simulink model "lunarMissionModel"  (R2022b)
settings: Solver=ode45  StartTime=0.0  StopTime=tf  RelTol=1e-12  AbsTol=1e-12
undefined symbols (not defined in the file): burnDuration, deltaVDRODeparture, deltaVDROInsertion, deltaVOPF, deltaVRPF, DRODepartureDirection, DROInsertionDirection, km, OPFDirection, RPFDirection, s, tDRODeparture, tDROInsertion, tOPF, tRPF
libraries: aerolibcelestial x1, aerolibconvert2 x1
settings Model: Creator=hsaranat  LastModifiedBy=hsaranat
settings SolverCC: AutoScaleAbsTol=off

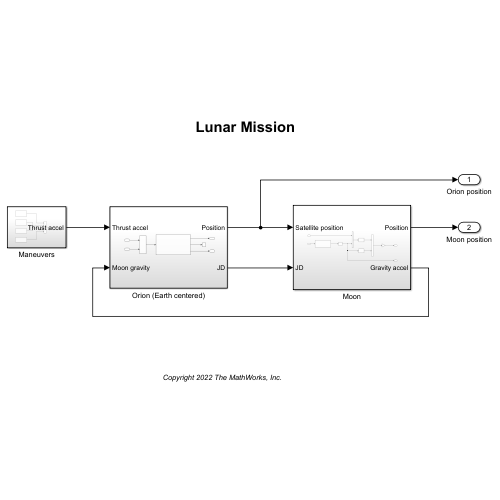
[thumbnail: Simulink's stored preview of the top-level diagram]
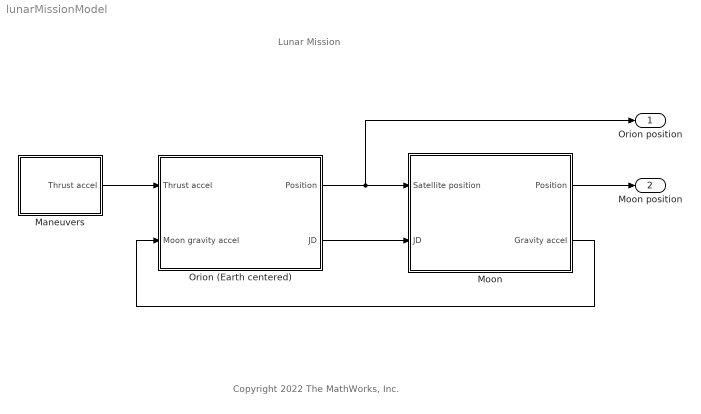
== system lunarMissionModel ==
  note: Lunar Mission
  note: Copyright 2022 The MathWorks, Inc.
  Maneuvers : Subsystem
  Moon : Subsystem
  Orion (Earth centered) : Subsystem
  Orion position : Outport
  Moon position : Outport  Port=2
  wires:
  Moon/1(Position) -> Moon position/1
  Orion (Earth centered)/2(JD) -> Moon/2(JD)
  Orion (Earth centered)/1(Position) -> Moon/1(Satellite position), Orion position/1
  Moon/2(Gravity accel) -> Orion (Earth centered)/2(Moon gravity accel)
  Maneuvers/1(Thrust accel) -> Orion (Earth centered)/1(Thrust accel)

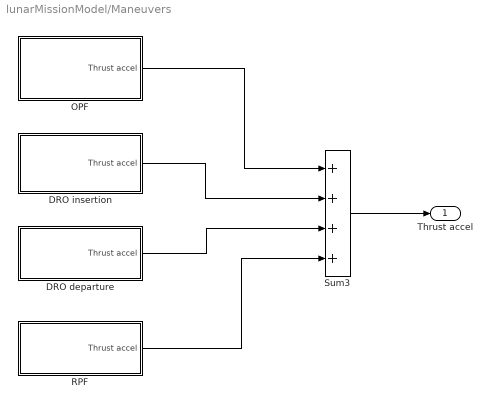
== system lunarMissionModel/Maneuvers ==
  DRO departure : Subsystem
  DRO insertion : Subsystem
  OPF : Subsystem
  RPF : Subsystem
  Sum3 : Sum  Inputs=++++
  Thrust accel : Outport
  wires:
  Sum3/1 -> Thrust accel/1
  OPF/1(Thrust accel) -> Sum3/1
  DRO insertion/1(Thrust accel) -> Sum3/2
  DRO departure/1(Thrust accel) -> Sum3/3
  RPF/1(Thrust accel) -> Sum3/4

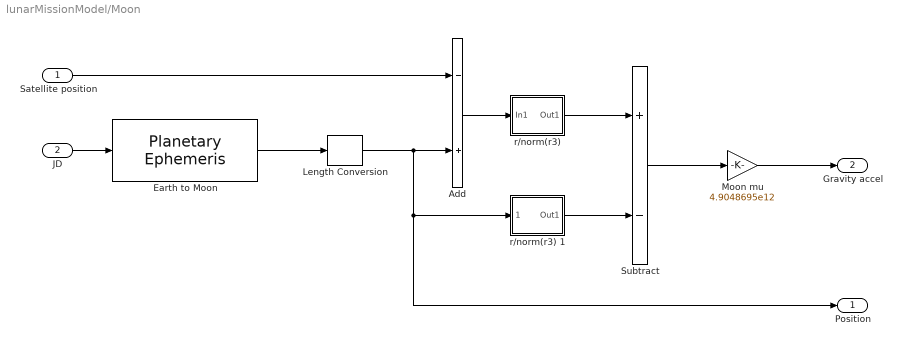
== system lunarMissionModel/Moon ==
  Satellite position : Inport
  JD : Inport  Port=2
  Add : Sum  Inputs=-+
  Earth to Moon : aerolibcelestial/Planetary Ephemeris  kmflag=km,km/s  epochflag=Julian date  de=DE405  nCenter=Earth  nTarget=Moon  errorflag=Error  velflag=off
  Length Conversion : aerolibconvert2/Length Conversion  IU=km  OU=m
  Moon mu : Gain  Gain=4.9048695e12
  Subtract : Sum  Inputs=+-
  r/norm(r3) : Subsystem
  r/norm(r3) 1 : Subsystem
  Position : Outport
  Gravity accel : Outport  Port=2
  wires:
  Earth to Moon/1 -> Length Conversion/1
  JD/1 -> Earth to Moon/1
  Length Conversion/1 -> Position/1, r/norm(r3) 1/1(1), Add/2
  r/norm(r3)/1(Out1) -> Subtract/1
  Moon mu/1 -> Gravity accel/1
  Satellite position/1 -> Add/1
  Add/1 -> r/norm(r3)/1(In1)
  r/norm(r3) 1/1(Out1) -> Subtract/2
  Subtract/1 -> Moon mu/1

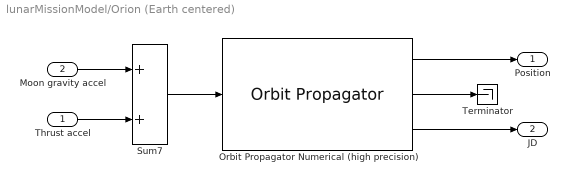
== system lunarMissionModel/Orion (Earth centered) ==
  Thrust accel : Inport
  Moon gravity accel : Inport  Port=2
  Orbit Propagator Numerical (high precision) : OrbitPropagator  propagator=Numerical (high precision)  accelIn=on  startDate=jd  action=None  stateFormatNum=ICRF state vector  eccentricity=0  inclination=30  raan=0  argPeriapsis=0  trueAnomaly=0  inertialPosition=initialPosition  inertialVelocity=initialVelocity  fixedPosition=[-4142689.0 -2676864.7 -4669861.6]  fixedVelocity=[1452.7 -6720.7 2568.1]  gravityModel=Point-mass  customR=3396200  customMu=4.305e13  customJ2=1.0826269e-03  customOmega=4.06125949e-3  useEOPs=off
  Sum7 : Sum
  Terminator : Terminator
  Position : Outport
  JD : Outport  Port=2
  wires:
  Orbit Propagator Numerical (high precision)/1 -> Position/1
  Orbit Propagator Numerical (high precision)/2 -> Terminator/1
  Sum7/1 -> Orbit Propagator Numerical (high precision)/1
  Orbit Propagator Numerical (high precision)/3 -> JD/1
  Thrust accel/1 -> Sum7/2
  Moon gravity accel/1 -> Sum7/1

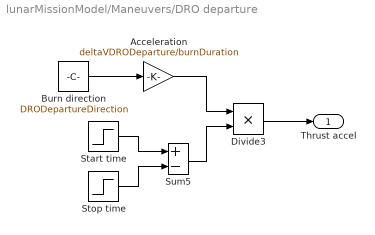
== system lunarMissionModel/Maneuvers/DRO departure ==
  Acceleration : Gain  Gain=deltaVDRODeparture/burnDuration
  Burn direction : Constant  Value=DRODepartureDirection
  Divide3 : Product  Inputs=**
  Start time : Step  Time=tDRODeparture  SampleTime=0
  Stop time : Step  Time=tDRODeparture+burnDuration  SampleTime=0
  Sum5 : Sum  Inputs=+-
  Thrust accel : Outport
  wires:
  Stop time/1 -> Sum5/2
  Burn direction/1 -> Acceleration/1
  Acceleration/1 -> Divide3/1
  Sum5/1 -> Divide3/2
  Start time/1 -> Sum5/1
  Divide3/1 -> Thrust accel/1

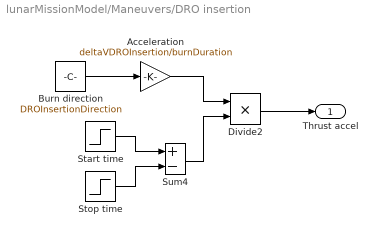
== system lunarMissionModel/Maneuvers/DRO insertion ==
  Acceleration : Gain  Gain=deltaVDROInsertion/burnDuration
  Burn direction : Constant  Value=DROInsertionDirection
  Divide2 : Product  Inputs=**
  Start time : Step  Time=tDROInsertion  SampleTime=0
  Stop time : Step  Time=tDROInsertion+burnDuration  SampleTime=0
  Sum4 : Sum  Inputs=+-
  Thrust accel : Outport
  wires:
  Acceleration/1 -> Divide2/1
  Start time/1 -> Sum4/1
  Divide2/1 -> Thrust accel/1
  Stop time/1 -> Sum4/2
  Sum4/1 -> Divide2/2
  Burn direction/1 -> Acceleration/1

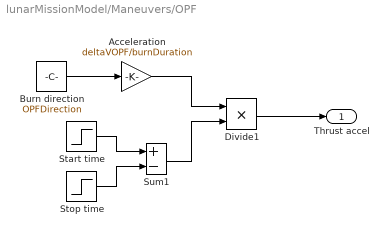
== system lunarMissionModel/Maneuvers/OPF ==
  Acceleration : Gain  Gain=deltaVOPF/burnDuration
  Burn direction : Constant  Value=OPFDirection
  Divide1 : Product  Inputs=**
  Start time : Step  Time=tOPF  SampleTime=0
  Stop time : Step  Time=tOPF+burnDuration  SampleTime=0
  Sum1 : Sum  Inputs=+-
  Thrust accel : Outport
  wires:
  Burn direction/1 -> Acceleration/1
  Sum1/1 -> Divide1/2
  Divide1/1 -> Thrust accel/1
  Acceleration/1 -> Divide1/1
  Start time/1 -> Sum1/1
  Stop time/1 -> Sum1/2

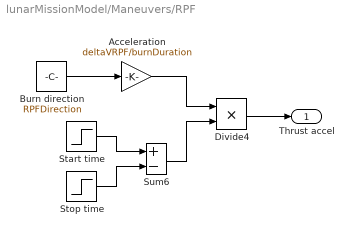
== system lunarMissionModel/Maneuvers/RPF ==
  Acceleration : Gain  Gain=deltaVRPF/burnDuration
  Burn direction : Constant  Value=RPFDirection
  Divide4 : Product  Inputs=**
  Start time : Step  Time=tRPF  SampleTime=0
  Stop time : Step  Time=tRPF+burnDuration  SampleTime=0
  Sum6 : Sum  Inputs=+-
  Thrust accel : Outport
  wires:
  Stop time/1 -> Sum6/2
  Acceleration/1 -> Divide4/1
  Sum6/1 -> Divide4/2
  Divide4/1 -> Thrust accel/1
  Start time/1 -> Sum6/1
  Burn direction/1 -> Acceleration/1

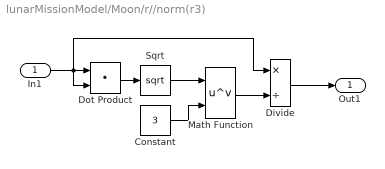
== system lunarMissionModel/Moon/r//norm(r3) ==
  In1 : Inport
  Constant : Constant  Value=3
  Divide : Product  Inputs=*/
  Dot Product : DotProduct  OutDataTypeStr=Inherit: Inherit via internal rule
  Math Function : Math  Operator=pow
  Sqrt : Sqrt
  Out1 : Outport
  wires:
  Divide/1 -> Out1/1
  Dot Product/1 -> Sqrt/1
  Sqrt/1 -> Math Function/1
  In1/1 -> Dot Product/1, Dot Product/2, Divide/1
  Constant/1 -> Math Function/2
  Math Function/1 -> Divide/2

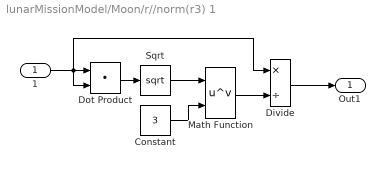
== system lunarMissionModel/Moon/r//norm(r3) 1 ==
  1 : Inport
  Constant : Constant  Value=3
  Divide : Product  Inputs=*/
  Dot Product : DotProduct  OutDataTypeStr=Inherit: Inherit via internal rule
  Math Function : Math  Operator=pow
  Sqrt : Sqrt
  Out1 : Outport
  wires:
  Math Function/1 -> Divide/2
  Constant/1 -> Math Function/2
  1/1 -> Divide/1, Dot Product/2, Dot Product/1
  Sqrt/1 -> Math Function/1
  Dot Product/1 -> Sqrt/1
  Divide/1 -> Out1/1
